simulink model "Inversor_Trifasico_Matlab_Pulsos_por_codigo"  (R2022a)
settings: Solver=ode4  StartTime=0.0  StopTime=0.1  FixedStep=0.0001  RelTol=1e-3
libraries: spsIGBTDiodeLib x6, spsVoltageMeasurementLib x4, spsSeriesRLCBranchLib x3, spsCurrentMeasurementLib x1, spsDCVoltageSourceLib x1, spsGroundLib x1, spspowerguiLib x1
settings Model: Creator=debian  LastModifiedBy=debian

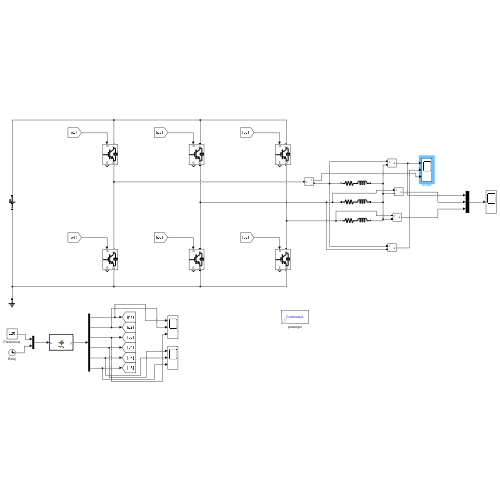
[thumbnail: Simulink's stored preview of the top-level diagram]
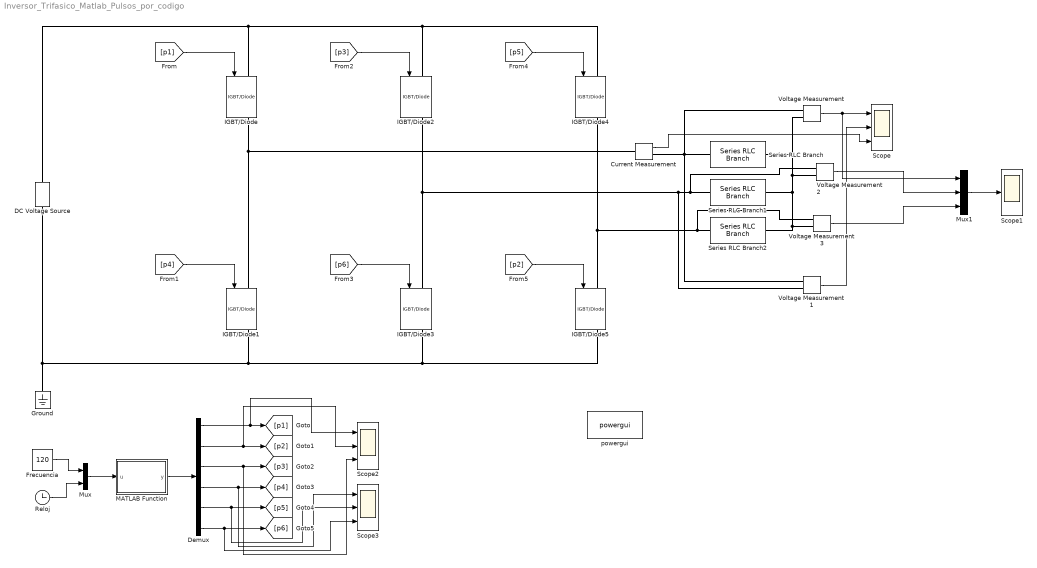
== system Inversor_Trifasico_Matlab_Pulsos_por_codigo ==
  Current Measurement : spsCurrentMeasurementLib/Current Measurement  PhasorSimulation=off  OutputType=Complex  PSBequivalent=0
  DC Voltage Source : spsDCVoltageSourceLib/DC Voltage Source  Amplitude=100  Measurements=None
  Demux : Demux  Outputs=6
  Frecuencia : Constant  Value=120
  Ground : spsGroundLib/Ground  LConnTagsString=a
  IGBT/Diode{,1..5} (6 alike) : spsIGBTDiodeLib/IGBT//Diode  Ron=1e-3  Rs=1e5  Cs=inf  Measurements=on
  MATLAB Function : MATLAB Function  TreatAsAtomicUnit=on
  Mux : Mux  Inputs=2
  Mux1 : Mux  Inputs=3
  Reloj : Clock
  Scope : Scope  NumInputPorts=3
  Scope1 : Scope
  Scope2 : Scope  NumInputPorts=3
  Scope3 : Scope  NumInputPorts=3
  Series RLC Branch : spsSeriesRLCBranchLib/Series RLC Branch  LConnTagsString=__new0  RConnTagsString=__new0  BranchType=RL  Resistance=10  Inductance=20e-3  SetiL0=off  InitialCurrent=0  Capacitance=1e-6  Setx0=off  InitialVoltage=0  Measurements=None
  Series RLC Branch1 : spsSeriesRLCBranchLib/Series RLC Branch  LConnTagsString=__new0  RConnTagsString=__new0  BranchType=RL  Resistance=10  Inductance=20e-3  SetiL0=off  InitialCurrent=0  Capacitance=1e-6  Setx0=off  InitialVoltage=0  Measurements=None
  Series RLC Branch2 : spsSeriesRLCBranchLib/Series RLC Branch  LConnTagsString=__new0  RConnTagsString=__new0  BranchType=RL  Resistance=10  Inductance=20e-3  SetiL0=off  InitialCurrent=0  Capacitance=1e-6  Setx0=off  InitialVoltage=0  Measurements=None
  Voltage Measurement{,1..3} (4 alike) : spsVoltageMeasurementLib/Voltage Measurement  PhasorSimulation=off  OutputType=Complex  PSBequivalent=0
  powergui : spspowerguiLib/powergui  Priority=1  SimulationMode=Continuous  SampleTime=50e-6  frequency=60  Iterations=50  frequencyindice=0  Pbase=100e6  ErrMax=1e-4  UnitsV=kV  UnitsW=MW  buscounter=0  FunctionMessages=off  echomessages=off  EnableUseOfTLC=off  CurrentSourceSwitches=off  DisableSnubberDevices=off  DisableRonSwitches=off  DisableVfSwitches=off  DisplayEquations=off  AutomaticDiscreteSolvers=off  SolverType=Tustin/Backward Euler (TBE)  Interpol=off  ExternalGateDelay=off  methode=off  Ts=100  x0status=blocks  SPID=on  SwTol=0  HookPort=off  NonlinearTolerance=1e-4  nMaxIteration=100  ContinueOnMaxIteration=off  RestoreLinks=warning  ResistiveCurrentMeasurement=off  Frange=[0:2:500]  Ylog=off  Xlog=on  ShowGrid=off  save=off  variable=ZData  structure=0  ZoomFFT=off  StartTime=0.0  cycles=1  DisplayStyle=1  fundamental=60  FreqAxis=off  MaxFrequency=1000  frequencyindicesteady=1  RmsSteady=1  display=off
  wires:
  [p1] -> IGBT/Diode/1
  [p4] -> IGBT/Diode1/1
  [p6] -> IGBT/Diode3/1
  [p3] -> IGBT/Diode2/1
  [p2] -> IGBT/Diode5/1
  [p5] -> IGBT/Diode4/1
  Frecuencia/1 -> Mux/1
  Reloj/1 -> Mux/2
  Mux/1 -> MATLAB Function/1(u)
  MATLAB Function/1(y) -> Demux/1
  Demux/1 -> Scope2/1, [p1]
  Demux/2 -> Scope2/2, [p2]
  Demux/3 -> Scope2/3, [p3]
  Demux/4 -> Scope3/1, [p4]
  Demux/5 -> Scope3/2, [p5]
  Demux/6 -> Scope3/3, [p6]
  Voltage Measurement/1 -> Mux1/1, Scope/1
  Voltage Measurement1/1 -> Scope/2
  Current Measurement/1 -> Scope/3
  Mux1/1 -> Scope1/1
  Voltage Measurement2/1 -> Mux1/2
  Voltage Measurement3/1 -> Mux1/3
  connections:
  DC Voltage Source/LConn1 -- IGBT/Diode1/RConn1 -- IGBT/Diode5/RConn1 -- IGBT/Diode3/RConn1 -- Ground/LConn1
  DC Voltage Source/RConn1 -- IGBT/Diode/LConn1 -- IGBT/Diode4/LConn1 -- IGBT/Diode2/LConn1
  IGBT/Diode5/LConn1 -- Voltage Measurement3/LConn1 -- Series RLC Branch2/LConn1 -- IGBT/Diode4/RConn1
  IGBT/Diode3/LConn1 -- Voltage Measurement2/LConn1 -- Series RLC Branch1/LConn1 -- Voltage Measurement1/LConn2 -- IGBT/Diode2/RConn1
  IGBT/Diode1/LConn1 -- Current Measurement/LConn1 -- IGBT/Diode/RConn1
  Series RLC Branch/RConn1 -- Voltage Measurement/LConn2 -- Series RLC Branch2/RConn1 -- Voltage Measurement3/LConn2 -- Series RLC Branch1/RConn1 -- Voltage Measurement2/LConn2
  Series RLC Branch/LConn1 -- Voltage Measurement1/LConn1 -- Current Measurement/RConn1 -- Voltage Measurement/LConn1

== matlab function Inversor_Trifasico_Matlab_Pulsos_por_codigo/MATLAB Function ==
  data: u input; y output
function y = fcn(u)

    f=u(1); %frecuencia
    w=2*pi*f; %frecuecnia angular
    t=u(2); %tiempo

    angulo=w*t; 
    CA=cos(angulo); %coseño del angulo
    SA=sin(angulo); %seno del angulo

    %las siguientes condiciones se usan para determinar un angulo entre 0 y
    %360°

    if SA>0&&CA>=0
        ang=asind(SA);
    elseif SA>0&&CA<=0
        ang=180-asind(SA);
    elseif SA<0&&CA<=0
        ang=180-(asind(SA));
    else
        ang=360+(asind(SA));
    end

    %Esquema de conmutacion de interruptores

    if(ang>0&&ang<=60)
        pulso1=1;
        pulso2=0;
        pulso3=0;
        pulso4=0;
        pulso5=1;
        pulso6=1;
    elseif(ang>60&&ang<=120)
        pulso1=1;
        pulso2=1;
        pulso3=0;
        pulso4=0;
        pulso5=0;
        pulso6=1;
    elseif(ang>120&&ang<=180)
        pulso1=1;
        pulso2=1;
        pulso3=1;
        pulso4=0;
        pulso5=0;
        pulso6=0;
    elseif(ang>180&&ang<=240)
        pulso1=0;
        pulso2=1;
        pulso3=1;
        pulso4=1;
        pulso5=0;
        pulso6=0;
    elseif(ang>240&&ang<=300)
        pulso1=0;
        pulso2=0;
        pulso3=1;
        pulso4=1;
        pulso5=1;
        pulso6=0;
    elseif(ang>300&&ang<=360)
        pulso1=0;
        pulso2=0;
        pulso3=0;
        pulso4=1;
        pulso5=1;
        pulso6=1;
    else
        pulso1=0;
        pulso2=0;
        pulso3=0;
        pulso4=0;
        pulso5=0;
        pulso6=0;
    end
y=[pulso1;pulso2;pulso3;pulso4;pulso5;pulso6];
